simulink library "holo_library"  (Simulink 7.0)
libraries: xbsIndex_r4 x53, casper_library x4
settings Model: Creator=Administrator  LastModifiedBy=Administrator

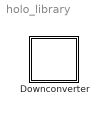
== system holo_library ==
  Downconverter : Subsystem

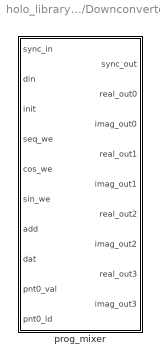
== system holo_library/Downconverter ==
  prog_mixer : Subsystem  mask{lookup_bits=9, coeff_bits=25, streams=4, din_bits=8, add_latency=1, bram_latency=2, mult_latency=2, numerator=1, denominator=8, offset=0, dout_bits=25, dout_bin_pt=24}
      mask prompts: lookup_bits "Lookup depth (2^?)"; coeff_bits "Coefficient resolution (bits)"; din_bits "Input data resolution (bits)"; add_latency "Adder latency"; bram_latency "BRAM latency"; mult_latency "Multiplier latency"; numerator "Numerator of preloaded frequency (N in N/Mxsampling frequency)"; denominator "Denominator of preloaded frequency (M in N/Mxsampling frequency)"; offset "Initial phase offset"; dout_bits "Output data bit width"; dout_bin_pt "Output data binary point"

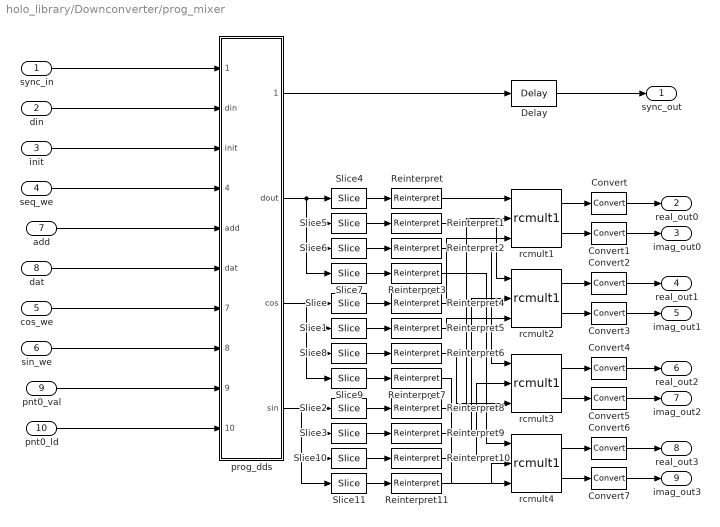
== system holo_library/Downconverter/prog_mixer ==
  sync_in : Inport  OutDataType=sfix(16)  OutScaling=2^0
  din : Inport  Port=2  OutDataType=sfix(16)  OutScaling=2^0
  init : Inport  Port=3  OutDataType=sfix(16)  OutScaling=2^0
  seq_we : Inport  Port=4  OutDataType=sfix(16)  OutScaling=2^0
  cos_we : Inport  Port=5  OutDataType=sfix(16)  OutScaling=2^0
  sin_we : Inport  Port=6  OutDataType=sfix(16)  OutScaling=2^0
  add : Inport  Port=7  OutDataType=sfix(16)  OutScaling=2^0
  dat : Inport  Port=8  OutDataType=sfix(16)  OutScaling=2^0
  pnt0_val : Inport  Port=9  OutDataType=sfix(16)  OutScaling=2^0
  pnt0_ld : Inport  Port=10  OutDataType=sfix(16)  OutScaling=2^0
  Convert{,1..7} (8 alike) : xbsIndex_r4/Convert  arith_type="Signed  (2's comp)"  n_bits=dout_bits  bin_pt=dout_bin_pt  quantization="Round  (unbiased: Even Values)"  overflow=Saturate  latency=1  dbl_ovrd=off  pipeline=off  block_type=convert
      settings: block_version=10.1.3
  Delay : xbsIndex_r4/Delay  en=off  latency=mult_latency+1  dbl_ovrd=off  reg_retiming=on  block_type=delay
      settings: block_version=11.4
  Reinterpret{,1..3} (4 alike) : xbsIndex_r4/Reinterpret  force_arith_type=on  arith_type="Signed  (2's comp)"  force_bin_pt=on  bin_pt=din_bits-1  block_type=reinterpret
      settings: infoedit="Changes signal type without altering the binary representation.   You can changed the signal between signed and unsigned, and relocate the binary point.<br><br>Hardware notes: In hardware this block costs nothing.<br><br>Example:  Suppose the input is 6 bits wide, signed, with 2 fractional bits, and the output is forced to unsigned with 0 fractional bits.  Then an input of -2.0 (1110.00 in binary 2's complement) becomes an output of 56 (111000 in binary)."
  Reinterpret{4..11} (8 alike) : xbsIndex_r4/Reinterpret  force_arith_type=on  arith_type="Signed  (2's comp)"  force_bin_pt=on  bin_pt=coeff_bits-2  block_type=reinterpret
      settings: infoedit="Changes signal type without altering the binary representation.   You can changed the signal between signed and unsigned, and relocate the binary point.<br><br>Hardware notes: In hardware this block costs nothing.<br><br>Example:  Suppose the input is 6 bits wide, signed, with 2 fractional bits, and the output is forced to unsigned with 0 fractional bits.  Then an input of -2.0 (1110.00 in binary 2's complement) becomes an output of 56 (111000 in binary)."
  Slice : xbsIndex_r4/Slice  nbits=coeff_bits  boolean_output=off  mode=Lower Bit Location + Width  bit1=0  base1=MSB of Input  bit0=coeff_bits*0  base0=LSB of Input  dbl_ovrd=off  block_type=slice
  Slice1 : xbsIndex_r4/Slice  nbits=coeff_bits  boolean_output=off  mode=Lower Bit Location + Width  bit1=0  base1=MSB of Input  bit0=coeff_bits*1  base0=LSB of Input  dbl_ovrd=off  block_type=slice
  Slice10 : xbsIndex_r4/Slice  nbits=coeff_bits  boolean_output=off  mode=Lower Bit Location + Width  bit1=0  base1=MSB of Input  bit0=coeff_bits*2  base0=LSB of Input  dbl_ovrd=off  block_type=slice
  Slice11 : xbsIndex_r4/Slice  nbits=coeff_bits  boolean_output=off  mode=Lower Bit Location + Width  bit1=0  base1=MSB of Input  bit0=coeff_bits*3  base0=LSB of Input  dbl_ovrd=off  block_type=slice
  Slice2 : xbsIndex_r4/Slice  nbits=coeff_bits  boolean_output=off  mode=Lower Bit Location + Width  bit1=0  base1=MSB of Input  bit0=coeff_bits*0  base0=LSB of Input  dbl_ovrd=off  block_type=slice
  Slice3 : xbsIndex_r4/Slice  nbits=coeff_bits  boolean_output=off  mode=Lower Bit Location + Width  bit1=0  base1=MSB of Input  bit0=coeff_bits*1  base0=LSB of Input  dbl_ovrd=off  block_type=slice
  Slice4 : xbsIndex_r4/Slice  nbits=din_bits  boolean_output=off  mode=Lower Bit Location + Width  bit1=0  base1=MSB of Input  bit0=din_bits*3  base0=LSB of Input  dbl_ovrd=off  block_type=slice
  Slice5 : xbsIndex_r4/Slice  nbits=din_bits  boolean_output=off  mode=Lower Bit Location + Width  bit1=0  base1=MSB of Input  bit0=din_bits*2  base0=LSB of Input  dbl_ovrd=off  block_type=slice
  Slice6 : xbsIndex_r4/Slice  nbits=din_bits  boolean_output=off  mode=Lower Bit Location + Width  bit1=0  base1=MSB of Input  bit0=din_bits*1  base0=LSB of Input  dbl_ovrd=off  block_type=slice
  Slice7 : xbsIndex_r4/Slice  nbits=din_bits  boolean_output=off  mode=Lower Bit Location + Width  bit1=0  base1=MSB of Input  bit0=din_bits*0  base0=LSB of Input  dbl_ovrd=off  block_type=slice
  Slice8 : xbsIndex_r4/Slice  nbits=coeff_bits  boolean_output=off  mode=Lower Bit Location + Width  bit1=0  base1=MSB of Input  bit0=coeff_bits*2  base0=LSB of Input  dbl_ovrd=off  block_type=slice
  Slice9 : xbsIndex_r4/Slice  nbits=coeff_bits  boolean_output=off  mode=Lower Bit Location + Width  bit1=0  base1=MSB of Input  bit0=coeff_bits*3  base0=LSB of Input  dbl_ovrd=off  block_type=slice
  prog_dds : Subsystem  mask(prog_dds){lookup_bits=lookup_bits, streams=streams, data_bits=coeff_bits, numerator=numerator, denominator=denominator, offset=offset, bram_latency=bram_latency}
      mask prompts: lookup_bits "Slowest frequency supported as fraction of sampling frequency (1/2^?)"; streams "Number of data streams"; data_bits "Resolution of mixing products (bits)"; numerator "Numerator of initial frequency (N in N/M*sampling frequency)"; denominator "Denominator of initial frequency (M in N/M*samping frequency)"; offset "Initial phase offset (samples)"; bram_latency "BRAM latency"
  rcmult1 : casper_library/Downconverter/mixer/rcmult1  SystemSampleTime=-1  latency=mult_latency
      link override Mult: precision=Full  arith_type="Signed  (2's comp)"  n_bits=8  bin_pt=2  quantization=Truncate  overflow=Wrap  en=off  latency=latency  dbl_ovrd=off  use_behavioral_HDL=on  opt=Speed  use_embedded=on  optimum_pipeline=off  pipeline=on  use_rpm=off  placement_style=Rectangular shape
      link override Mult: infoedit=Hardware notes: To check for the optimum internal pipeline stages of the dedicated multiplier you must select 'Test for optimum pipelining'.<br><br>Optimization Goal: For implementation into device fabric (LUTs), the Speed or Area optimization will take effect only if it's supported by IP for the particular device family. Otherwise, the results will be identical regardless of the selection.  xl_area=[0, 0, 0, 0, 0, 0, 0]
  rcmult2 : casper_library/Downconverter/mixer/rcmult1  SystemSampleTime=-1  latency=mult_latency
      link override Mult: precision=Full  arith_type="Signed  (2's comp)"  n_bits=8  bin_pt=2  quantization=Truncate  overflow=Wrap  en=off  latency=latency  dbl_ovrd=off  use_behavioral_HDL=on  opt=Speed  use_embedded=on  optimum_pipeline=off  pipeline=on  use_rpm=off  placement_style=Rectangular shape
      link override Mult: infoedit=Hardware notes: To check for the optimum internal pipeline stages of the dedicated multiplier you must select 'Test for optimum pipelining'.<br><br>Optimization Goal: For implementation into device fabric (LUTs), the Speed or Area optimization will take effect only if it's supported by IP for the particular device family. Otherwise, the results will be identical regardless of the selection.  xl_area=[0, 0, 0, 0, 0, 0, 0]
  rcmult3 : casper_library/Downconverter/mixer/rcmult1  SystemSampleTime=-1  latency=mult_latency
      link override Mult: precision=Full  arith_type="Signed  (2's comp)"  n_bits=8  bin_pt=2  quantization=Truncate  overflow=Wrap  en=off  latency=latency  dbl_ovrd=off  use_behavioral_HDL=on  opt=Speed  use_embedded=on  optimum_pipeline=off  pipeline=on  use_rpm=off  placement_style=Rectangular shape
      link override Mult: infoedit=Hardware notes: To check for the optimum internal pipeline stages of the dedicated multiplier you must select 'Test for optimum pipelining'.<br><br>Optimization Goal: For implementation into device fabric (LUTs), the Speed or Area optimization will take effect only if it's supported by IP for the particular device family. Otherwise, the results will be identical regardless of the selection.  xl_area=[0, 0, 0, 0, 0, 0, 0]
  rcmult4 : casper_library/Downconverter/mixer/rcmult1  SystemSampleTime=-1  latency=mult_latency
      link override Mult: precision=Full  arith_type="Signed  (2's comp)"  n_bits=8  bin_pt=2  quantization=Truncate  overflow=Wrap  en=off  latency=latency  dbl_ovrd=off  use_behavioral_HDL=on  opt=Speed  use_embedded=on  optimum_pipeline=off  pipeline=on  use_rpm=off  placement_style=Rectangular shape
      link override Mult: infoedit=Hardware notes: To check for the optimum internal pipeline stages of the dedicated multiplier you must select 'Test for optimum pipelining'.<br><br>Optimization Goal: For implementation into device fabric (LUTs), the Speed or Area optimization will take effect only if it's supported by IP for the particular device family. Otherwise, the results will be identical regardless of the selection.  xl_area=[0, 0, 0, 0, 0, 0, 0]
  sync_out : Outport  OutDataType=sfix(16)  OutScaling=2^0
  real_out0 : Outport  Port=2  OutDataType=sfix(16)  OutScaling=2^0
  imag_out0 : Outport  Port=3  OutDataType=sfix(16)  OutScaling=2^0
  real_out1 : Outport  Port=4  OutDataType=sfix(16)  OutScaling=2^0
  imag_out1 : Outport  Port=5  OutDataType=sfix(16)  OutScaling=2^0
  real_out2 : Outport  Port=6  OutDataType=sfix(16)  OutScaling=2^0
  imag_out2 : Outport  Port=7  OutDataType=sfix(16)  OutScaling=2^0
  real_out3 : Outport  Port=8  OutDataType=sfix(16)  OutScaling=2^0
  imag_out3 : Outport  Port=9  OutDataType=sfix(16)  OutScaling=2^0
  wires:
  Convert7/1 -> imag_out3/1
  Convert6/1 -> real_out3/1
  Convert5/1 -> imag_out2/1
  Convert4/1 -> real_out2/1
  Convert3/1 -> imag_out1/1
  Convert2/1 -> real_out1/1
  Convert1/1 -> imag_out0/1
  Convert/1 -> real_out0/1
  din/1 -> prog_dds/2(din)
  Slice4/1 -> Reinterpret/1
  Slice5/1 -> Reinterpret1/1
  Slice6/1 -> Reinterpret2/1
  Slice7/1 -> Reinterpret3/1
  Slice/1 -> Reinterpret4/1
  Slice1/1 -> Reinterpret5/1
  Slice8/1 -> Reinterpret6/1
  Slice9/1 -> Reinterpret7/1
  Slice2/1 -> Reinterpret8/1
  Slice3/1 -> Reinterpret9/1
  Slice10/1 -> Reinterpret10/1
  Slice11/1 -> Reinterpret11/1
  prog_dds/2(dout) -> Slice4/1, Slice5/1, Slice6/1, Slice7/1
  Reinterpret/1 -> rcmult1/1
  prog_dds/3(cos) -> Slice/1, Slice9/1, Slice8/1, Slice1/1
  prog_dds/4(sin) -> Slice2/1, Slice3/1, Slice11/1, Slice10/1
  Reinterpret1/1 -> rcmult2/1
  Reinterpret2/1 -> rcmult3/1
  prog_dds/1(sync_out) -> Delay/1
  Delay/1 -> sync_out/1
  rcmult1/1 -> Convert/1
  rcmult1/2 -> Convert1/1
  rcmult2/1 -> Convert2/1
  rcmult2/2 -> Convert3/1
  rcmult3/1 -> Convert4/1
  rcmult3/2 -> Convert5/1
  rcmult4/1 -> Convert6/1
  rcmult4/2 -> Convert7/1
  sync_in/1 -> prog_dds/1(sync_in)
  init/1 -> prog_dds/3(init)
  seq_we/1 -> prog_dds/4(seq_we)
  add/1 -> prog_dds/5(add)
  dat/1 -> prog_dds/6(dat)
  cos_we/1 -> prog_dds/7(cos_we)
  sin_we/1 -> prog_dds/8(sin_we)
  pnt0_val/1 -> prog_dds/9(pnt0_val)
  pnt0_ld/1 -> prog_dds/10(pnt0_ld)
  Reinterpret3/1 -> rcmult4/1
  Reinterpret4/1 -> rcmult1/3
  Reinterpret5/1 -> rcmult2/3
  Reinterpret6/1 -> rcmult3/3
  Reinterpret7/1 -> rcmult4/3
  Reinterpret8/1 -> rcmult1/2
  Reinterpret9/1 -> rcmult2/2
  Reinterpret10/1 -> rcmult3/2
  Reinterpret11/1 -> rcmult4/2

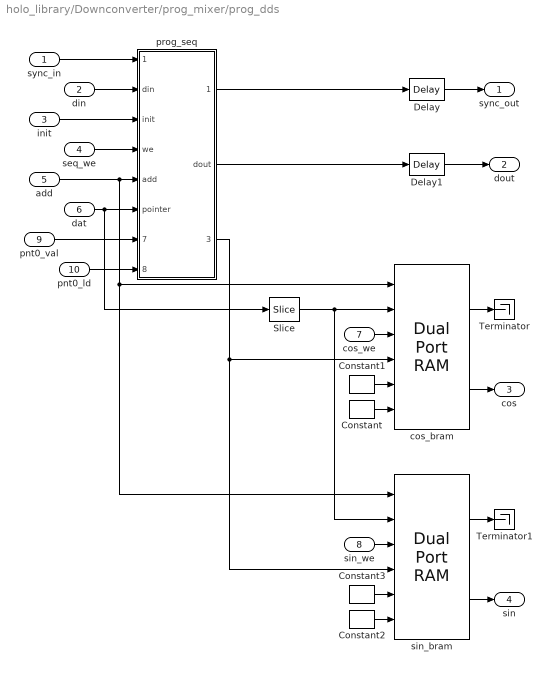
== system holo_library/Downconverter/prog_mixer/prog_dds ==
  sync_in : Inport  OutDataType=sfix(16)  OutScaling=2^0
  din : Inport  Port=2  OutDataType=sfix(16)  OutScaling=2^0
  init : Inport  Port=3  OutDataType=sfix(16)  OutScaling=2^0
  seq_we : Inport  Port=4  OutDataType=sfix(16)  OutScaling=2^0
  add : Inport  Port=5  OutDataType=sfix(16)  OutScaling=2^0
  dat : Inport  Port=6  OutDataType=sfix(16)  OutScaling=2^0
  cos_we : Inport  Port=7  OutDataType=sfix(16)  OutScaling=2^0
  sin_we : Inport  Port=8  OutDataType=sfix(16)  OutScaling=2^0
  pnt0_val : Inport  Port=9  OutDataType=sfix(16)  OutScaling=2^0
  pnt0_ld : Inport  Port=10  OutDataType=sfix(16)  OutScaling=2^0
  Constant : xbsIndex_r4/Constant  arith_type=Boolean  const=0  n_bits=16  bin_pt=14  explicit_period=off  period=1  equ=P=C  opselect=C  inp2=PCIN>>17  opr=+  inp1=P  carry=CIN  dbl_ovrd=off  block_type=constant
      settings: block_version=11.4
  Constant1 : xbsIndex_r4/Constant  arith_type=Unsigned  const=0  n_bits=streams*data_bits  bin_pt=0  explicit_period=off  period=1  equ=P=C  opselect=C  inp2=PCIN>>17  opr=+  inp1=P  carry=CIN  dbl_ovrd=off  block_type=constant
      settings: block_version=11.4
  Constant2 : xbsIndex_r4/Constant  arith_type=Boolean  const=0  n_bits=16  bin_pt=14  explicit_period=off  period=1  equ=P=C  opselect=C  inp2=PCIN>>17  opr=+  inp1=P  carry=CIN  dbl_ovrd=off  block_type=constant
      settings: block_version=11.4
  Constant3 : xbsIndex_r4/Constant  arith_type=Unsigned  const=0  n_bits=streams*data_bits  bin_pt=0  explicit_period=off  period=1  equ=P=C  opselect=C  inp2=PCIN>>17  opr=+  inp1=P  carry=CIN  dbl_ovrd=off  block_type=constant
      settings: block_version=11.4
  Delay : xbsIndex_r4/Delay  en=off  latency=bram_latency  dbl_ovrd=off  reg_retiming=on  block_type=delay
      settings: block_version=11.4
  Delay1 : xbsIndex_r4/Delay  en=off  latency=bram_latency  dbl_ovrd=off  reg_retiming=on  block_type=delay
      settings: block_version=11.4
  Slice : xbsIndex_r4/Slice  nbits=data_bits  boolean_output=off  mode=Lower Bit Location + Width  bit1=0  base1=MSB of Input  bit0=0  base0=LSB of Input  dbl_ovrd=off  block_type=slice
  Terminator : Terminator
  Terminator1 : Terminator
  cos_bram : xbsIndex_r4/Dual Port RAM  depth=(2^lookup_bits)*streams  initVector=[mod( cos((mod(floor([0:denominator*streams-1]/streams) + mod([0:denominator*streams-1],streams)*numerator, denominator) * 2 * pi)/denominator) * 2^(data_bits-2) + 2^data_bits, 2^data_bits), zeros(1,(2^lookup_bits*streams)-(denominator*streams))]  distributed_mem=Block RAM  init_a=0  init_b=0  rst_a=off  rst_b=off  en_a=off  en_b=off  latency=bram_latency  write_mode_A=Read After Write  write_mode_B=Read After Write  dbl_ovrd=off  optimize=Speed  use_rpm=on  block_type=dpram
      settings: block_version=11.4
  prog_seq : Subsystem  mask(prog_seq){pnt_bits=lookup_bits, pre_pnt_vec=[mod([0:denominator-1]+(numerator*streams), denominator), zeros(1,2^lookup_bits-denominator)], pre_init_pnt=offset}
      mask prompts: pnt_bits "Max number pointers  (2^?)"; pre_pnt_vec "Preloaded pointer vector"; pre_init_pnt "Preloaded initial pointer"
      mask help:
      | Generates a preloaded sequence of vectors. Each vector contains a pointer to the next in the sequence.
      | add - vector target address used during programming
      | pointer - address of next vector in sequence
      | vec0_pnt -
      | init - starts the sequence
  sin_bram : xbsIndex_r4/Dual Port RAM  depth=(2^lookup_bits)*streams  initVector=[mod( -sin((mod(floor([0:denominator*streams-1]/streams) + mod([0:denominator*streams-1],streams)*numerator, denominator) * 2 * pi)/denominator) * 2^(data_bits-2) + 2^data_bits, 2^data_bits), zeros(1,(2^lookup_bits*streams)-(denominator*streams))]  distributed_mem=Block RAM  init_a=0  init_b=0  rst_a=off  rst_b=off  en_a=off  en_b=off  latency=bram_latency  write_mode_A=Read After Write  write_mode_B=Read After Write  dbl_ovrd=off  optimize=Speed  use_rpm=on  block_type=dpram
      settings: block_version=11.4
  sync_out : Outport  OutDataType=sfix(16)  OutScaling=2^0
  dout : Outport  Port=2  OutDataType=sfix(16)  OutScaling=2^0
  cos : Outport  Port=3  OutDataType=sfix(16)  OutScaling=2^0
  sin : Outport  Port=4  OutDataType=sfix(16)  OutScaling=2^0
  wires:
  sync_in/1 -> prog_seq/1(sync_in)
  din/1 -> prog_seq/2(din)
  init/1 -> prog_seq/3(init)
  seq_we/1 -> prog_seq/4(we)
  add/1 -> cos_bram/1, sin_bram/1, prog_seq/5(add)
  dat/1 -> Slice/1, prog_seq/6(pointer)
  cos_we/1 -> cos_bram/3
  prog_seq/1(sync_out) -> Delay/1
  Delay/1 -> sync_out/1
  Delay1/1 -> dout/1
  Slice/1 -> cos_bram/2, sin_bram/2
  prog_seq/3(location) -> cos_bram/4, sin_bram/4
  Constant/1 -> cos_bram/6
  cos_bram/1 -> Terminator/1
  Constant1/1 -> cos_bram/5
  cos_bram/2 -> cos/1
  sin_bram/1 -> Terminator1/1
  sin_bram/2 -> sin/1
  sin_we/1 -> sin_bram/3
  Constant3/1 -> sin_bram/5
  Constant2/1 -> sin_bram/6
  pnt0_val/1 -> prog_seq/7(pnt0_val)
  pnt0_ld/1 -> prog_seq/8(pnt0_ld)
  prog_seq/2(dout) -> Delay1/1

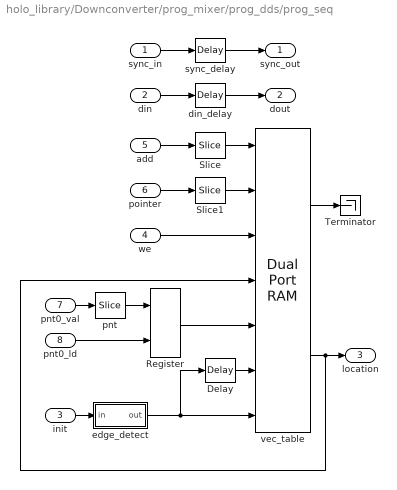
== system holo_library/Downconverter/prog_mixer/prog_dds/prog_seq ==
  sync_in : Inport  OutDataType=sfix(16)  OutScaling=2^0
  din : Inport  Port=2  OutDataType=sfix(16)  OutScaling=2^0
  init : Inport  Port=3  OutDataType=sfix(16)  OutScaling=2^0
  we : Inport  Port=4  OutDataType=sfix(16)  OutScaling=2^0
  add : Inport  Port=5  OutDataType=sfix(16)  OutScaling=2^0
  pointer : Inport  Port=6  OutDataType=sfix(16)  OutScaling=2^0
  pnt0_val : Inport  Port=7  OutDataType=sfix(16)  OutScaling=2^0
  pnt0_ld : Inport  Port=8  OutDataType=sfix(16)  OutScaling=2^0
  Delay : xbsIndex_r4/Delay  en=off  latency=1  dbl_ovrd=off  reg_retiming=off  block_type=delay
      settings: block_version=11.4
  Register : xbsIndex_r4/Register  init=pre_pnt_vec(1)  rst=off  en=on  dbl_ovrd=off  block_type=register
      settings: block_version=11.4
  Slice : xbsIndex_r4/Slice  nbits=pnt_bits  boolean_output=off  mode=Lower Bit Location + Width  bit1=0  base1=MSB of Input  bit0=0  base0=LSB of Input  dbl_ovrd=off  block_type=slice
  Slice1 : xbsIndex_r4/Slice  nbits=pnt_bits  boolean_output=off  mode=Lower Bit Location + Width  bit1=0  base1=MSB of Input  bit0=0  base0=LSB of Input  dbl_ovrd=off  block_type=slice
  Terminator : Terminator
  din_delay : xbsIndex_r4/Delay  en=off  latency=2  dbl_ovrd=off  reg_retiming=on  block_type=delay
      settings: block_version=11.4
  edge_detect : Subsystem  AncestorBlock=casper_library/Misc/edge_detect  mask(edge_detect){edge=Rising, polarity=Active High, x_in=[0 0.08 0.08 0.16 0.16 0.24 0.24 0.32 0.32 0.4], y_in=[-1 -1  1  1  1  1  1  1  1  1], x_out=[0.6 0.68 0.68 0.76 0.76 0.84 0.84 0.92 0.92 1], y_out=[-1 -1  1  1 -1 -1 -1 -1 -1 -1]}
      mask prompts: edge "Edge Type"; polarity "Output Polarity"; x_in "Input X Positions"; y_in "Input Y Positions"; x_out "Output X Positions"; y_out "Output Y Positions"
      mask help: Output is active for one-cycle after each edge of the specified type (i.e. rising, falling or both).
      mask init:
      | edge_detect_init(gcb,...
      |     'edge',edge,...
      |     'polarity',polarity,...
      |     'x_in',x_in,...
      |     'x_out',x_out,...
      |     'y_in',y_in,...
      |     'y_out',y_out);
      | 
      | x_in_num=str2num(getfield(getfield(get_param(gcb,'UserData'),'parameters'),'x_in'));
      | x_out_num=str2num(getfield(getfield(get_param(gcb,'UserData'),'parameters'),'x_out'));
      | y_in_num=str2num(getfield(getfield(get_param(gcb,'UserData'),'parameters'),'y_in'));
      | y_out_num=str2num(getfield(getfield(get_param(gcb,'UserData'),'parameters'),'y_out'));
      settings: AttributesFormatString=|
      | rising edges
      | active high
      mask Help: Output is active for one-cycle after each edge of the specified type (i.e. rising, falling, or both).  Latency is zero.
      mask StyleString: popup(Rising|Falling|Both),popup(Active High|Active Low),edit,edit,edit,edit
      mask Display:
      | plot(x_in_num,0.5+y_in_num*0.2);
      | plot(x_out_num,0.5+y_out_num*0.2);
  pnt : xbsIndex_r4/Slice  nbits=pnt_bits  boolean_output=off  mode=Lower Bit Location + Width  bit1=0  base1=MSB of Input  bit0=0  base0=LSB of Input  dbl_ovrd=off  block_type=slice
  sync_delay : xbsIndex_r4/Delay  en=off  latency=2  dbl_ovrd=off  reg_retiming=on  block_type=delay
      settings: block_version=11.4
  vec_table : xbsIndex_r4/Dual Port RAM  depth=2^pnt_bits  initVector=[pre_init_pnt, pre_pnt_vec(2:2^pnt_bits)]  distributed_mem=Block RAM  init_a=0  init_b=0  rst_a=off  rst_b=on  en_a=off  en_b=off  latency=1  write_mode_A=Read Before Write  write_mode_B=Read Before Write  dbl_ovrd=off  optimize=Speed  use_rpm=on  block_type=dpram
      settings: block_version=11.4
  sync_out : Outport  OutDataType=sfix(16)  OutScaling=2^0
  dout : Outport  Port=2  OutDataType=sfix(16)  OutScaling=2^0
  location : Outport  Port=3  OutDataType=sfix(16)  OutScaling=2^0
  wires:
  Slice/1 -> vec_table/1
  vec_table/2 -> location/1, vec_table/4
  vec_table/1 -> Terminator/1
  init/1 -> edge_detect/1(in)
  edge_detect/1(out) -> Delay/1, vec_table/7
  Delay/1 -> vec_table/6
  add/1 -> Slice/1
  pnt0_val/1 -> pnt/1
  we/1 -> vec_table/3
  pointer/1 -> Slice1/1
  sync_delay/1 -> sync_out/1
  sync_in/1 -> sync_delay/1
  din/1 -> din_delay/1
  din_delay/1 -> dout/1
  Slice1/1 -> vec_table/2
  pnt/1 -> Register/1
  Register/1 -> vec_table/5
  pnt0_ld/1 -> Register/2

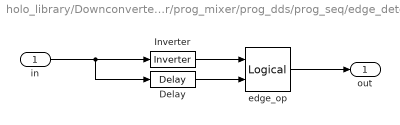
== system holo_library/Downconverter/prog_mixer/prog_dds/prog_seq/edge_detect ==
  in : Inport  OutDataType=sfix(16)  OutScaling=2^0
  Delay : xbsIndex_r4/Delay  en=off  latency=1  dbl_ovrd=off  reg_retiming=off  block_type=delay
      settings: xl_area=[0, 0, 0, 0, 0, 0, 0]
  Inverter : xbsIndex_r4/Inverter  en=off  latency=0  dbl_ovrd=off  block_type=inv
      settings: xl_area=[0, 0, 0, 0, 0, 0, 0]
  edge_op : xbsIndex_r4/Logical  logical_function=NOR  inputs=2  en=off  latency=0  precision=Full  arith_type=Unsigned  n_bits=8  bin_pt=2  align_bp=on  dbl_ovrd=off  block_type=logical
      settings: xl_area=[0, 0, 0, 0, 0, 0, 0]
  out : Outport  OutDataType=sfix(16)  OutScaling=2^0
  wires:
  Delay/1 -> edge_op/2
  in/1 -> Delay/1, Inverter/1
  edge_op/1 -> out/1
  Inverter/1 -> edge_op/1
